simulink model "nonlinear_lqg_controller"  (R2021a)
settings: Solver=VariableStepAuto  StartTime=0.0  StopTime=100  RelTol=1e-3
undefined symbols (not defined in the file): C, K, sysKF
settings Model: Creator=savna  LastModifiedBy=savna

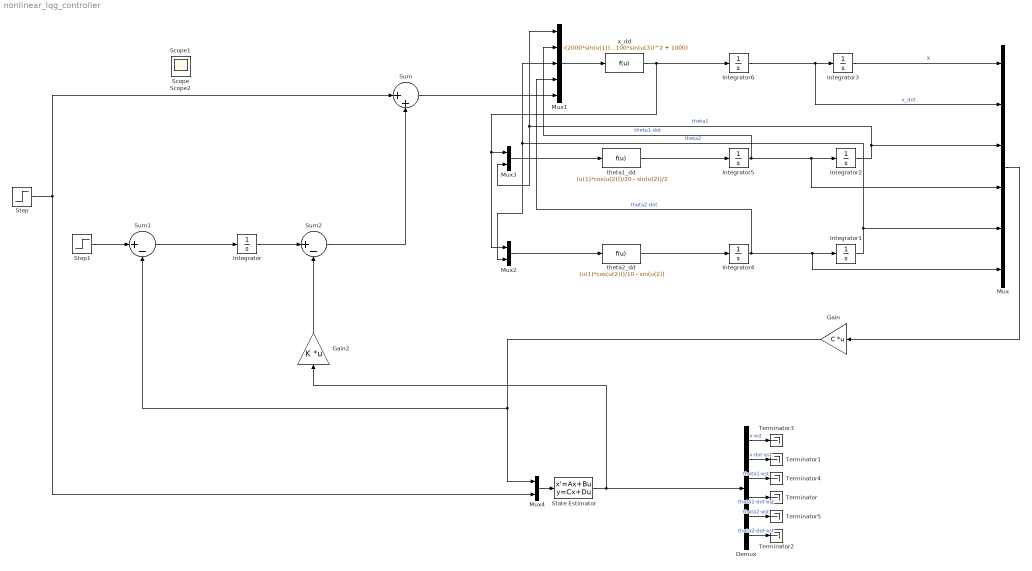
== system nonlinear_lqg_controller ==
  Demux : Demux  Outputs=6
  Gain : Gain  Gain=C  Multiplication=Matrix(K*u)
  Gain2 : Gain  Gain=K  Multiplication=Matrix(K*u)
  Integrator{,4..6} (4 alike) : Integrator
  Integrator1 : Integrator  InitialCondition=0.1
  Integrator2 : Integrator  InitialCondition=0.1
  Integrator3 : Integrator  InitialCondition=0.5
  Mux : Mux  Inputs=6
  Mux1 : Mux  Inputs=5
  Mux2 : Mux  Inputs=2
  Mux3 : Mux  Inputs=2
  Mux4 : Mux  Inputs=2
  "State Estimator " : StateSpace  A=sysKF.a  B=sysKF.b  C=sysKF.c  D=sysKF.d  InitialCondition=0
  Step : Step  SampleTime=5
  Step1 : Step  SampleTime=5
  Sum : Sum  Inputs=|++
  Sum1 : Sum  Inputs=|+-
  Sum2 : Sum  Inputs=|+-
  Terminator{,1..5} (6 alike) : Terminator
  theta1_dd : Fcn  Expr=(u(1)*cos(u(2)))/20 - sin(u(2))/2
  theta2_dd : Fcn  Expr=(u(1)*cos(u(2)))/10 - sin(u(2))
  x_dd : Fcn  Expr=-(2000*sin(u(1))*u(2)^2 + 1000*sin(u(3))*u(4)^2 - u(5) + 1000*cos(u(1))*sin(u(1)) - 1000*cos(u(3))*sin(u(3)))/(100*sin(u(1))^2 + 100*sin(u(3))^2 + 1000)
  Scope : Scope
  Scope1 : Scope
  Scope2 : Scope
  wires:
  Sum2/1 -> Sum/2
  Demux/2 -> Terminator1/1  "x-dot-est"
  Demux/4 -> Terminator/1  "theta1-dot-est"
  Step/1 -> Mux4/2, Sum/1
  Gain2/1 -> Sum2/2
  "State Estimator "/1 -> Gain2/1, Demux/1
  Sum1/1 -> Integrator/1
  Demux/6 -> Terminator2/1  "theta2-dot-est"
  Integrator/1 -> Sum2/1
  Gain/1 -> Mux4/1, Sum1/2
  Step1/1 -> Sum1/1
  Mux4/1 -> "State Estimator "/1
  Integrator2/1 -> Mux3/2, Mux1/1, Mux/3  "theta1"
  Integrator1/1 -> Mux2/2, Mux1/3, Mux/5  "theta2"
  theta1_dd/1 -> Integrator5/1
  Mux1/1 -> x_dd/1
  theta2_dd/1 -> Integrator4/1
  Integrator5/1 -> Mux1/2, Mux/4, Integrator2/1  "theta1-dot"
  x_dd/1 -> Mux2/1, Mux3/1, Integrator6/1
  Mux2/1 -> theta2_dd/1
  Integrator4/1 -> Mux1/4, Integrator1/1, Mux/6  "theta2-dot"
  Mux3/1 -> theta1_dd/1
  Integrator3/1 -> Mux/1  "X"
  Integrator6/1 -> Mux/2, Integrator3/1  "x_dot"
  Mux/1 -> Gain/1
  Sum/1 -> Mux1/5
  Demux/1 -> Terminator3/1  "x-est"
  Demux/3 -> Terminator4/1  "theta1-est"
  Demux/5 -> Terminator5/1  "theta2-est"
